simulink model "Estimator"  (Simulink 10.1)
settings: Solver=FixedStepDiscrete  StartTime=0.0  StopTime=3  FixedStep=Ts  RelTol=1e-3
PreLoadFcn:
  | Ts=1e-3;
libraries: dspsrcs4 x4, dspbuff3 x2, dspobslib x2, dspswit3 x1
settings Model: Creator=Carchesion  LastModifiedBy=upattacini
settings DataIOCC: SignalLoggingSaveFormat=ModelDataLogs  SaveOutput=off  SignalLogging=off  SaveTime=off
settings OptimizationCC: ExpressionDepthLimit=2147483647  InitFltsAndDblsToZero=on
settings DebuggingCC: SolverPrmCheckMsg=warning  FcnCallInpInsideContextMsg=warning  StateNameClashWarn=warning
settings SFSimCC: SimParseCustomCode=off

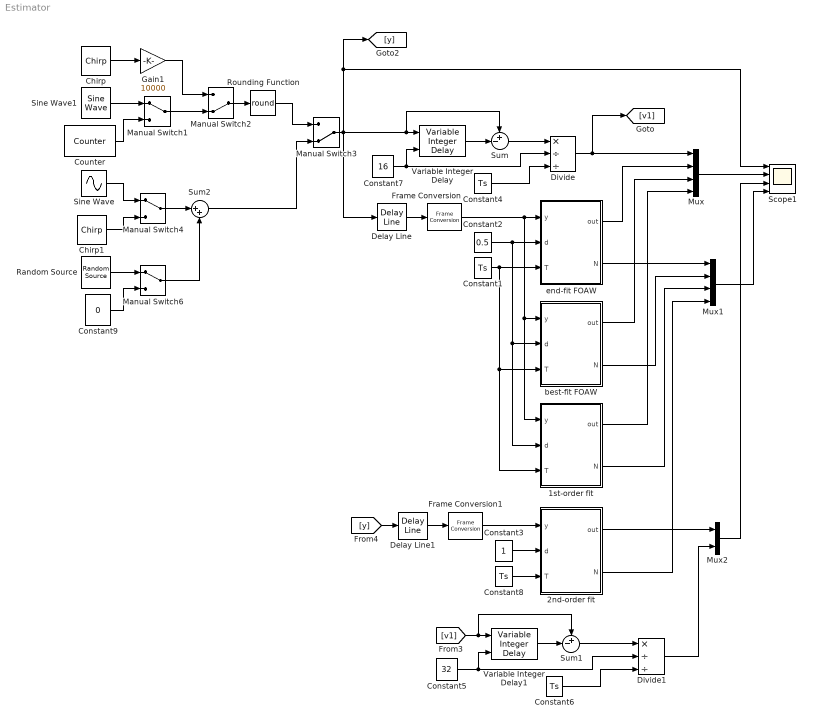
== system Estimator ==
  1st-order fit : MATLAB Function  TreatAsAtomicUnit=on
  2nd-order fit : MATLAB Function  TreatAsAtomicUnit=on
  Chirp : dspsrcs4/Chirp  sweep=Linear  mode=Bidirectional  f0=0  f1=5  t1=1  Tsweep=1  phase=0  Ts=Ts  spf=1  datatype=Double  OutputFrames=on
  Chirp1 : dspsrcs4/Chirp  sweep=Linear  mode=Bidirectional  f0=0  f1=10  t1=1  Tsweep=1  phase=0  Ts=Ts  spf=1  datatype=Double  OutputFrames=on
  Constant{1,4,6,8} (4 alike) : Constant  Value=Ts
  Constant2 : Constant  Value=0.5
  Constant3 : Constant
  Constant5 : Constant  Value=32
  Constant7 : Constant  Value=16
  Constant9 : Constant  Value=0
  Counter : dspswit3/Counter  Direction=Up  CountEvent=Free running  CounterSize=32 bits  MaxCount=255  InitialCount=0  Output=Count  HitValue=32  ResetInput=off  SamplesPerFrame=1  Ts=Ts  CntDtype=double  HitDtype=Logical
  Delay Line : dspbuff3/Delay Line  siz=16  ic=0  directfeed=off  enable_output=off  hold_output=off  OutputFrames=on
      settings: SourceProductBaseCode=DS
  Delay Line1 : dspbuff3/Delay Line  siz=32  ic=0  directfeed=off  enable_output=off  hold_output=off  OutputFrames=on
      settings: SourceProductBaseCode=DS
  Divide : Product  Inputs=*//
  Divide1 : Product  Inputs=*//
  Frame Conversion : FrameConversion  OutFrame=Sample-based
  Frame Conversion1 : FrameConversion  OutFrame=Sample-based
  Gain1 : Gain  Gain=10000
  Manual Switch1 : ManualSwitch
  Manual Switch2 : ManualSwitch  CurrentSetting=0
  Manual Switch3 : ManualSwitch  CurrentSetting=0
  Manual Switch4 : ManualSwitch
  Manual Switch6 : ManualSwitch
  Mux : Mux
  Mux1 : Mux
  Mux2 : Mux  Inputs=2
  Random Source : dspsrcs4/Random Source  SrcType=Gaussian  NormMethod=Ziggurat  CltLength=12  MinVal=0  MaxVal=1  MeanVal=0  VarVal=1e-4  RepMode=Not repeatable  rawSeed=1  IsInherit=off  SampMode=Discrete  SampTime=Ts  SampFrame=1  DataType=Double  OutComplex=Real  OutputFrames=on
  Rounding Function : Rounding  Operator=round
  Scope1 : Scope  NumInputPorts=4
  Sine Wave : Sin  Frequency=2*pi*5  SampleTime=Ts
  Sine Wave1 : dspsrcs4/Sine Wave  Amplitude=10  Frequency=0.1  Phase=0  SampleMode=Discrete  OutComplex=Real  CompMethod=Trigonometric fcn  TableSize=Speed  SampleTime=Ts  SamplesPerFrame=1  ResetState=Restart at time zero  OutputFrames=on  dataType=double  wordLen=16  udDataType=sfix(16)  fracBitsMode=Best precision  numFracBits=15  OutDataTypeStr=double  LastOutDataTypeStr=double
  Sum : Sum  Inputs=+-|
  Sum1 : Sum  Inputs=+-|
  Sum2 : Sum  Inputs=|++
  Variable Integer Delay : dspobslib/Variable Integer Delay  dmax=1024  InputProcessing=Columns as channels (frame based)  ic=0  noDFT=off
      settings: SourceProductBaseCode=DS
  Variable Integer Delay1 : dspobslib/Variable Integer Delay  dmax=1024  InputProcessing=Columns as channels (frame based)  ic=0  noDFT=off
      settings: SourceProductBaseCode=DS
  best-fit FOAW : MATLAB Function  TreatAsAtomicUnit=on
  end-fit FOAW : MATLAB Function  TreatAsAtomicUnit=on
  wires:
  Counter/1 -> Manual Switch1/2
  Sine Wave1/1 -> Manual Switch1/1
  Delay Line/1 -> Frame Conversion/1
  Constant1/1 -> end-fit FOAW/3(T), best-fit FOAW/3(T), 1st-order fit/3(T)
  Constant2/1 -> end-fit FOAW/2(d), best-fit FOAW/2(d), 1st-order fit/2(d)
  Mux/1 -> Scope1/2
  end-fit FOAW/2(N) -> Mux1/1
  best-fit FOAW/2(N) -> Mux1/2
  best-fit FOAW/1(out) -> Mux/3
  Manual Switch3/1 -> Delay Line/1, Variable Integer Delay/1, Sum/1, Scope1/1, [y]
  Frame Conversion/1 -> end-fit FOAW/1(y), best-fit FOAW/1(y), 1st-order fit/1(y)
  Manual Switch1/1 -> Manual Switch2/2
  Manual Switch2/1 -> Rounding Function/1
  Chirp/1 -> Gain1/1
  Gain1/1 -> Manual Switch2/1
  Variable Integer Delay/1 -> Sum/2
  Constant7/1 -> Variable Integer Delay/2, Divide/2
  Sum/1 -> Divide/1
  Divide/1 -> [v1], Mux/1
  Constant4/1 -> Divide/3
  1st-order fit/2(N) -> Mux1/3
  2nd-order fit/2(N) -> Mux1/4
  Mux1/1 -> Scope1/4
  [v1] -> Sum1/1, Variable Integer Delay1/1
  Variable Integer Delay1/1 -> Sum1/2
  Constant5/1 -> Variable Integer Delay1/2, Divide1/2
  Sum1/1 -> Divide1/1
  Constant6/1 -> Divide1/3
  Divide1/1 -> Mux2/2
  Mux2/1 -> Scope1/3
  2nd-order fit/1(out) -> Mux2/1
  Constant3/1 -> 2nd-order fit/2(d)
  Delay Line1/1 -> Frame Conversion1/1
  Frame Conversion1/1 -> 2nd-order fit/1(y)
  [y] -> Delay Line1/1
  Constant8/1 -> 2nd-order fit/3(T)
  Rounding Function/1 -> Manual Switch3/1
  Sine Wave/1 -> Manual Switch4/1
  Manual Switch4/1 -> Sum2/1
  Random Source/1 -> Manual Switch6/1
  Constant9/1 -> Manual Switch6/2
  Manual Switch6/1 -> Sum2/2
  Chirp1/1 -> Manual Switch4/2
  Sum2/1 -> Manual Switch3/2
  1st-order fit/1(out) -> Mux/4
  end-fit FOAW/1(out) -> Mux/2

== matlab function best-fit FOAW ==
  data: y input double; out output double; d input double; T input double; N output double
function [out,N]=fcn(y,d,T)

L=length(y);
bn=0;

for N=1:L-1
    an=y(L-N);
    bn=0;
    for i=0:N
        bn=bn+(N-2*i)*y(L-i);
    end
    bn=bn/(T*N*(N+1)*(N+2)/6);
    
    finish=false;
    for i=1:N-1
        Ly=an+bn*(N-i)*T;
        if abs(y(L-i)-Ly)>d
            finish=true;
            break;
        end
    end
    
    if finish
        break;
    end
end

out=bn;

== matlab function end-fit FOAW ==
  data: y input double; out output double; d input double; T input double; N output double
function [out,N]=fcn(y,d,T)

L=length(y);
bn=0;

for N=1:L-1
    an=y(L-N);
    bn=(y(L)-y(L-N))/(N*T);

    finish=false;
    for i=1:N-1
        Ly=an+bn*(N-i)*T;
        if abs(y(L-i)-Ly)>d
            finish=true;
            break;
        end
    end
    
    if finish
        break;
    end
end

out=bn;

== matlab function 1st-order fit ==
  data: y input double; out output double; d input double; T input double; N output double
function [out,N]=fcn(y,d,T)
%#ok<*NASGU>

coder.extrinsic('polyfitHelper');

persistent n;
if isempty(n)
    n=1;
end

L=length(y);
pos=zeros(1,2);
Ly=0;
N=n;

for j=max(1,n-1):min(n+1,L-1)
    pos=polyfitHelper(y,1,T,j);

    finish=false;
    for i=0:j
        Ly=polyval(pos,i*T);
        if abs(y(L-j+i)-Ly)>d
            finish=true;
            break;
        end
    end
    
    if finish
        N=j;
        break;
    end
    N=j;
end

out=pos(1);
n=N;

== matlab function 2nd-order fit ==
  data: y input double; out output double; d input double; T input double; N output double
function [out,N]=fcn(y,d,T)
%#ok<*NASGU>

coder.extrinsic('polyfitHelper');

persistent n;
if isempty(n)
    n=1;
end

L=length(y);
pos=zeros(1,3);
v=0;                
a=0;
Ly=0;
N=n;

for j=max(2,n-1):min(n+1,L-1)    
    pos=polyfitHelper(y,2,T,j);

    finish=false;
    for i=0:j
        Ly=polyval(pos,i*T);
        if abs(y(L-j+i)-Ly)>d
            finish=true;
            break;
        end
    end
    
    if finish
        N=j;
        break;
    end
    N=j;
end

out=2*pos(1);
n=N;
